simulink model "Hybrid_P2_Parallel_ETE"  (R2017b)
settings: Solver=FixedStepAuto  StartTime=0.0  StopTime=length(Speed)  FixedStep=0.01  MaxStep=0.01  RelTol=1e-3  EnableMultiTasking=on
PostLoadFcn:
  | , if any(exist('dsrtsu_mdlpostloadfcn', 'file') == [2, 3, 6]), try dsrtsu_mdlpostloadfcn('Execute', bdroot); catch fprintf('Error in PostLoadFcn (dsrtsu_mdlpostloadfcn) for model "%s":\n %s\n', bdroot, lasterr); end, end,
undefined symbols (not defined in the file): Actuators, APP1_OOR, APP2_OOR, APP_Mismatch, Brk_Flt, cal, ClutchEngag, CycLength, CycNmb, DiscIntNeverNeededParam, eng, Engine, EngOverTemp, ENGTRQ_MSMCH_Degraded_CP, ENGTRQ_MSMCH_ErrCritical_CP, ENGTRQ_MSMCH_LimpHome_CP, EngTrqMismatch, ess, ESSOverTemp, gb, Gearbox, KeyPos_Flt, lib_Actuators, lib_EMachine_2017a, lib_Sensors_2017a, Loss, LossCAN, Machine, MCUOverTemp, mot, MotDirMismatch, MotOverTemp, MotTrqMismatch, PRNDL_Flt, Ratio, RegenFault, Scope_new, Scopes1, Sensors, Spd, StopIndex, t_amb, time, tloop
libraries: simulink x117, EC2_libraries x9, powerlib_meascontrol x2, CalculationGallon x1, lib_Chassis x1, lib_DCDC x1, lib_Differential x1, lib_HVESS x1, lib_Engine x1, lib_OBC x1, lib_Transmission x1, Transmission_Validation x1
(part 1 of 10)
settings Model: DSRTSU_INTERNAL_RTI_VER=480  DSRTSU_INTERNAL_RTI_TYPE=rti1006  RTICANMMDATA=struct('GeneralSetupData',struct('modelroot','D:\EcoCAR3\Controls\HIL\Y3\P2_Parallel_MIL_Model','generalsettings',struct('filesettings',struct('destfolder',struct('Name','RTICANMM_FILES','Check',1),'buildfolder',struct('Name','.','Check',1),'AbsDestfolder',struct('Name','D:\EcoCAR3\Controls\HIL\Y3\P2_Parallel_MIL_Model\RTICANMM_FILES'),'AbsBuildfolder',struct('Name','D:\EcoCAR3\Controls\HIL\Y3\P2_Parallel_MIL_Model'))),'options',struct('addpaths',1,'rmpaths',1,'addtrcexclusion',logical(1),'cannavigator',struct('checkmonitoring',0),'show_usrtrc',0,'use_usrtrc',0),'advanced',struct('options',[1 1 1 1 1 1 1 1 1 1 1 1 1 1 1 1 1 1 1 1 1 1 1 1 1 1 1 1 1 1 1 1 1 1 1 1 1 1 1 1 1 1 1 1 1 1 1 1 1 1 1 1 1 1 1 1 1 1 1 1 1 1 1 1 1 1 1 1 1 1 1 1 1 1 1 1 1 1 1 1 1 1 1 1 1 1 1 1 1 1 1 1 1 1 1 1 1 1 1 1]),'MPSetup',{{}},'modelname','P2_Parallel_MIL_02_16_2017','block','P2_Parallel_MIL_02_16_2017'))  DSRTSU_INTERNAL_RTIFPGA=70  SimulationMode=accelerator  Creator=EcoCar  LastModifiedBy=Lyu19
settings SolverCC: ExtrapolationOrder=1  NumberNewtonIterations=4
settings OptimizationCC: BlockReduction=off  OptimizeBlockIOStorage=off  BufferReuse=off  GlobalBufferReuse=off  ExpressionFolding=off  LocalBlockOutputs=off  EfficientMapNaN2IntZero=off
settings DebuggingCC: AllowSymbolicDim=off  NonBusSignalsTreatedAsBus=warning  SFUnexpectedBacktrackingDiag=warning  SFNoUnconditionalDefaultTransitionDiag=warning  SFExecutionAtInitializationDiag=none
settings HardwareCC: ProdBitPerPointer=32  ProdBitPerSizeT=32  ProdBitPerPtrDiffT=32  ProdLargestAtomicInteger=Integer  ProdWordSize=32  ProdHWDeviceType=Custom Processor->Custom  TargetBitPerPointer=64  TargetBitPerSizeT=64  TargetBitPerPtrDiffT=64  TargetLongLongMode=on  TargetIntDivRoundTo=Zero  TargetEndianess=LittleEndian  TargetWordSize=64  TargetHWDeviceType=MATLAB Host  ProdEqTarget=off
settings ModelReferenceCC: PropagateSignalLabelsOutOfModel=off
settings CodeAppCC: MaxIdLength=128  StateflowObjectComments=on
settings GRTTargetCC: TargetLangStandard=C89/C90 (ANSI)  CombineOutputUpdateFcns=off  GRTInterface=on
settings ConfigComp: CovMetricSettings=dw  CovHtmlReporting=on  CovSaveCumulativeToWorkspaceVar=on  CovSaveSingleToWorkspaceVar=on  CovExternalEMLEnable=off
settings SimscapeCC: SimscapeNormalizeSystem=off

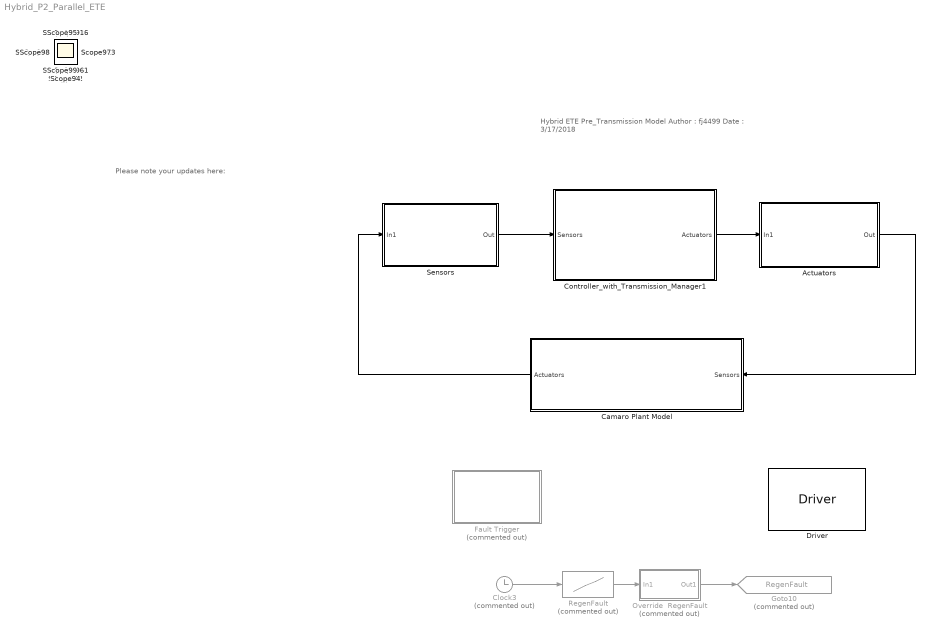
== system Hybrid_P2_Parallel_ETE ==
  note: Please note your updates here:
  note: Hybrid ETE Pre_Transmission Model
      |
      | Author : fj4499
      | Date : 3/17/2018
  Actuators : Subsystem  AncestorBlock=lib_Actuators/Actuators
  Camaro Plant Model : Subsystem
      mask Display: image('Images/Vehicle.jpg')
  Clock3 : Clock  Commented=on
  Controller_with_Transmission_Manager1 : Subsystem
      mask Display: image('Images/HCU.jpg')
  Driver : lib_Driver/Driver  SystemSampleTime=-1
      link override Driver Control/Regen3: Value=0
  "Fault Trigger " : Subsystem  Commented=on  mask(Fault Trigger){Mismatch_APP_ON=on, APP1_OOR_ON=on, APP2_OOR_ON=on, Brk_Flt_ON=on, KeyPos_Flt_ON=on, PRNDL_Flt_ON=on, LossCAN_ON=on, MotTrqMismatch_ON=on, MotDirMismatch_ON=on, EngTrqMismatch_ON=on, MotOverTemp_ON=on, MCUOverTemp_ON=on, EngOverTemp_ON=on, ESSOverTemp_ON=on, ClutchEngagFlt=on}
      mask help:
      | Check the box: override the fault (Control Port value=1;)
      | Uncheck the box: Implement the fault (Control Port value=0;)
      mask DialogControl DriverInterfaceFault Prompt: Driver Interface Fault
      mask DialogControl Container3 Prompt: Component Fault
      mask Display:
      | plot([1 2 2.01 3 4], [0 0 1 1 1]);
      | disp('           Fault Trigger')
  Goto10 : Goto  Commented=on  GotoTag=RegenFault  TagVisibility=global
  Override  RegenFault : Subsystem  Commented=on
  RegenFault : Lookup  Commented=on  InputValues=time  Table=RegenFault  LookUpMeth=Interpolation-Use End Values  OutDataTypeStr=int8
  Sensors : Subsystem  AncestorBlock=lib_Sensors_2017a/Sensors
  Scope{,1..146} (147 alike) : Scope
  wires:
  Clock3/1 -> RegenFault/1
  RegenFault/1 -> Override  RegenFault/1(In1)
  Override  RegenFault/1(Out1) -> Goto10/1
  Controller_with_Transmission_Manager1/1(Actuators) -> Actuators/1(In1)
  Actuators/1(Out) -> Camaro Plant Model/1(Sensors)
  Camaro Plant Model/1(Actuators) -> Sensors/1(In1)
  Sensors/1(Out) -> Controller_with_Transmission_Manager1/1(Sensors)

== system Hybrid_P2_Parallel_ETE/Actuators ==
  In1 : Inport
  Analog : Subsystem
  Bus Creator : BusCreator  Inputs=3
  CAN : Subsystem
  Digital : Subsystem
  Memory : Memory  InheritSampleTime=on
  Out : Outport
  wires:
  In1/1 -> CAN/1(In1), Analog/1(In1), Digital/1(In1)
  Bus Creator/1 -> Memory/1
  Digital/1(Out1) -> Bus Creator/3  "Digital"
  CAN/1(Out1) -> Bus Creator/1  "CAN"
  Analog/1(Out1) -> Bus Creator/2  "Analog"
  Memory/1 -> Out/1

== system Hybrid_P2_Parallel_ETE/Camaro Plant Model ==
  Sensors : Inport
  Add : Sum  Inputs=+++
      mask Display:
      | port_label('input',1,'+');
      | port_label('input',2,'+');
      | port_label('input',3,'+');
  Bus Creator : BusCreator  Inputs=3
  Bus Creator1 : BusCreator  Inputs=7
  Bus Creator2 : BusCreator  Inputs=1
  Bus Selector : BusSelector  OutputSignals=Analog,CAN.to VEH_CAN,CAN.to EBCAN,CAN.to HV_CAN,Digital
  Calculate MPGe : Subsystem  Commented=on
  Calculate MPGe1 : CalculationGallon/Calculate MPGe
  Chassis : lib_Chassis/Chassis  SystemSampleTime=-1
      link override Grade: InputValues=time
  DC-DC Converter : lib_DCDC/DC-DC Converter  SystemSampleTime=-1
  Differential : lib_Differential/Differential  SystemSampleTime=-1
      settings: SourceProductName=The database C:\Users\vrajm\AppData\Roaming\MathWorks\MATLAB\R2017b\slblocks_master.db is locked, or a table in the database is locked. (database is locked)
  E-Machine : Subsystem  AncestorBlock=lib_EMachine_2017a/E-Machine
      mask Display:
      | image('Images/motor.png')
      | color('red');
      | port_label('Input',1,'Volt');
      | port_label('Input',2,'ShaftIn');
      | port_label('Input',3,'SpdOut');
      | port_label('Output',1,'Crr');
      | port_label('Output',2,'ShaftOut');
      | port_label('Output',3,'SpdIn');
  ESS : lib_HVESS/ESS  SystemSampleTime=-1
  Ground : Ground
  ICE Simple1 : lib_Engine/ICE Simple1  SystemSampleTime=-1
  On-Board Charger : lib_OBC/On-Board Charger  SystemSampleTime=-1
      settings: SourceProductName=The database C:\Users\vrajm\AppData\Roaming\MathWorks\MATLAB\R2017b\slblocks_master.db is locked, or a table in the database is locked. (database is locked)
  Scopes : Subsystem  Commented=on
      mask Display: image('Images/Scope.jpg')
  Scopes1 : Subsystem  AncestorBlock=Scope_new/Scopes1
      mask Display: image('Images/Scope.jpg')
  Transmission : Subsystem  AncestorBlock=lib_Transmission/Transmission
      mask Display:
      | image('Images\Trans.png')
      | color('red');
      | port_label('Input',1,'ShaftIn')
      | port_label('Input',2,'SpdOut')
      | port_label('Output',1,'ShaftOut')
      | port_label('Output',2,'SpdIn')
  Transmission Validation Results : Transmission_Validation/Transmission Validation Results  Commented=on  SystemSampleTime=-1
  Wheels : lib_Wheels/Wheels  SystemSampleTime=-1
      link override Grade: InputValues=time
      settings: SourceProductName=The database C:\Users\vrajm\AppData\Roaming\MathWorks\MATLAB\R2017b\slblocks_master.db is locked, or a table in the database is locked. (database is locked)
  Actuators : Outport
  tag scope: Analog=global, Digital=global, HCU_to_EBCAN=global, HCU_to_HV_CAN=global, HCU_to_VEH_CAN=global
  wires:
  Differential/1 -> Wheels/1
  Wheels/1 -> Chassis/1
  Chassis/1 -> Wheels/2
  Differential/2 -> Transmission/2(SpdOut)
  Transmission/1(ShaftOut) -> Differential/1
  ESS/1 -> DC-DC Converter/1, E-Machine/1(voltage), On-Board Charger/1
  DC-DC Converter/1 -> Add/3
  On-Board Charger/1 -> Add/2
  Add/1 -> ESS/1
  Transmission/2(SpdIn) -> E-Machine/3(Mot_SpdOut)
  E-Machine/2(Motor_ShaftOut) -> Transmission/1(ShaftIn)
  E-Machine/1(current) -> Add/1
  Bus Creator/1 -> Actuators/1
  Sensors/1 -> Bus Selector/1
  Bus Selector/1 -> [Analog]  "<Analog>"
  Bus Selector/2 -> [HCU_to_VEH_CAN]  "<to VEH_CAN>"
  Bus Selector/3 -> [HCU_to_EBCAN]  "<to EBCAN>"
  Bus Selector/4 -> [HCU_to_HV_CAN]  "<to HV_CAN>"
  Bus Selector/5 -> [Digital]  "<Digital>"
  Wheels/2 -> Differential/2
  E-Machine/3(Motor_SpdIn) -> ICE Simple1/1
  [ECM_to_HCU] -> Bus Creator1/1
  [TCM_to_HCU] -> Bus Creator1/2
  [BCM_to_HCU] -> Bus Creator1/3
  [BMS_to_HCU] -> Bus Creator1/4
  [MCU_to_HCU] -> Bus Creator1/5
  Bus Creator2/1 -> Bus Creator1/6  "APM_to_HCU"
  [OBC_to_HCU] -> Bus Creator1/7
  Bus Creator1/1 -> Bus Creator/1  "CAN"
  [Driver_Request] -> Bus Creator/2  "Driver_Signals"
  [DCDC_to_HCU] -> Bus Creator/3
  Ground/1 -> Bus Creator2/1  "APM_CAN"
  ICE Simple1/1 -> E-Machine/2(Mot_ShaftIn)

== system Hybrid_P2_Parallel_ETE/Controller_with_Transmission_Manager1 ==
  Sensors : Inport
  HSC : Subsystem
  Actuators : Outport
  wires:
  HSC/1(Actuators) -> Actuators/1
  Sensors/1 -> HSC/1(Sensors)

== system Hybrid_P2_Parallel_ETE/Fault Trigger  ==
  Clock3 : Clock
  Component Diagnostics setting : Subsystem
  Driver Interface Diagnostics setting : Subsystem
  wires:
  Clock3/1 -> Component Diagnostics setting/1(time), Driver Interface Diagnostics setting/1(time)

== system Hybrid_P2_Parallel_ETE/Override  RegenFault ==
  note: This subsystem is used to override the model value of a signal to a constant value
  note: Override Switch Subsystem
  In1 : Inport
  Constant : Constant  Value=0
  Multiport Switch : MultiPortSwitch  DataPortOrder=Zero-based contiguous  Inputs=2
  Signal Override Switch 0 = Use Model 1 = Use Constant : Constant  Value=0
  Out1 : Outport
  wires:
  Signal Override Switch 0 = Use Model 1 = Use Constant/1 -> Multiport Switch/1
  In1/1 -> Multiport Switch/2
  Multiport Switch/1 -> Out1/1
  Constant/1 -> Multiport Switch/3

== system Hybrid_P2_Parallel_ETE/Sensors ==
  In1 : Inport
  Analog : Subsystem
  Bus Creator : BusCreator  Inputs=3
  Bus Selector : BusSelector  OutputSignals=CAN
  CAN : Subsystem
  Digital : Subsystem
  Out : Outport
  wires:
  Bus Creator/1 -> Out/1
  In1/1 -> Digital/1(In1), Analog/1(In1), Bus Selector/1
  Bus Selector/1 -> CAN/1(In1)  "<CAN>"
  CAN/1(Out1) -> Bus Creator/1  "from_CAN"
  Analog/1(Out1) -> Bus Creator/2  "from_Analog"
  Digital/1(Out1) -> Bus Creator/3  "from_Digital"

== system Hybrid_P2_Parallel_ETE/Actuators/Analog ==
  In1 : Inport
  Bus Creator : BusCreator  Inputs=1
  Bus Selector : BusSelector  OutputSignals=Controls.EngAppReq
  Data Type Conversion : DataTypeConversion
  Out1 : Outport
  wires:
  In1/1 -> Bus Selector/1
  Bus Creator/1 -> Out1/1
  Bus Selector/1 -> Data Type Conversion/1  "<EngAppReq>"
  Data Type Conversion/1 -> Bus Creator/1  "EngAppReq"

== system Hybrid_P2_Parallel_ETE/Actuators/CAN ==
  In1 : Inport
  Bus Creator : BusCreator  Inputs=3
  EBCAN : Subsystem
  HV_CAN : Subsystem
  VEH_CAN : Subsystem
  Out1 : Outport
  wires:
  VEH_CAN/1(Out1) -> Bus Creator/1  "to VEH_CAN"
  EBCAN/1(Out1) -> Bus Creator/2  "to EBCAN"
  HV_CAN/1(Out1) -> Bus Creator/3  "to HV_CAN"
  Bus Creator/1 -> Out1/1
  In1/1 -> HV_CAN/1(In1), EBCAN/1(In1), VEH_CAN/1(In1)

== system Hybrid_P2_Parallel_ETE/Actuators/Digital ==
  In1 : Inport
  Bus Creator : BusCreator  Inputs=8
  Bus Selector : BusSelector  OutputSignals=BMS_Digital.T_15,BMS_Digital.T_30,BMS_Digital.T_30C,Fuel_Pump_Control.Pump_Commands.FuelPump_Disable,OBC_Digital.Brusa_Enable,Axiomatic_CAN.GFD_Light,Axiomatic_CAN.HV_Chg_Light,Axiomatic_CAN.Veh_Ready_Light
  Data Type Conversion : DataTypeConversion
  Data Type Conversion1 : DataTypeConversion
  Out1 : Outport
  wires:
  In1/1 -> Bus Selector/1
  Bus Creator/1 -> Out1/1  "Digital"
  Bus Selector/4 -> Bus Creator/4  "<FuelPump_Disable>"
  Bus Selector/3 -> Bus Creator/3  "<T_30C>"
  Bus Selector/2 -> Data Type Conversion1/1  "<T_30>"
  Bus Selector/1 -> Data Type Conversion/1  "<T_15>"
  Bus Selector/5 -> Bus Creator/5  "<Brusa_Enable>"
  Bus Selector/6 -> Bus Creator/6  "<GFD_Light>"
  Bus Selector/7 -> Bus Creator/7  "<HV_Chg_Light>"
  Bus Selector/8 -> Bus Creator/8  "<Veh_Ready_Light>"
  Data Type Conversion/1 -> Bus Creator/1  "T_15"
  Data Type Conversion1/1 -> Bus Creator/2  "T_30"

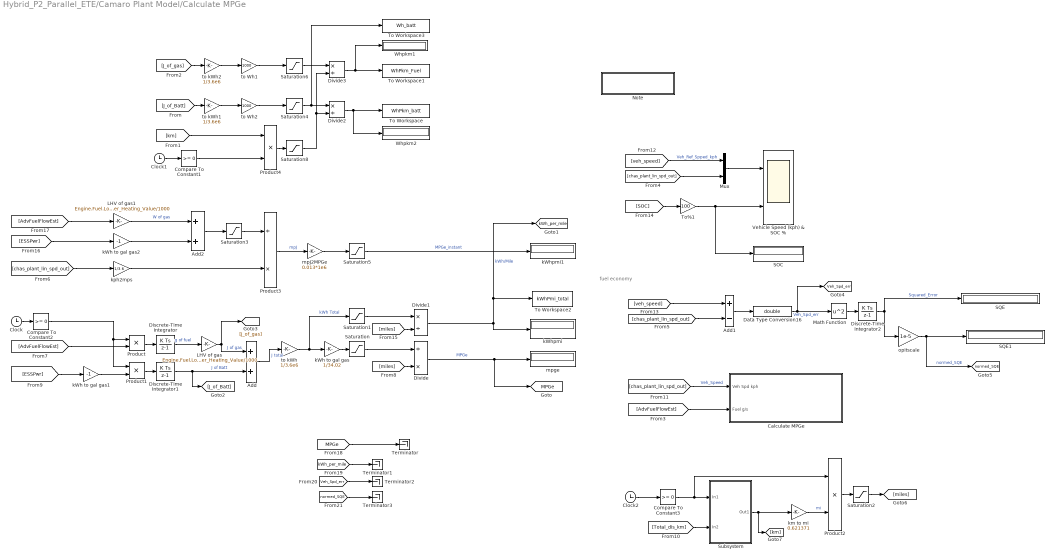
== system Hybrid_P2_Parallel_ETE/Camaro Plant Model/Calculate MPGe ==
  note: fuel economy
  Add : Sum
  Add1 : Sum  Inputs=+-
  Add2 : Sum
  Calculate MPGe : Subsystem
  Clock : Clock
  Clock1 : Clock
  Clock2 : Clock
  Compare To Constant1 : simulink/Logic and Bit Operations/Compare To Constant  relop=>=  const=0  OutDataTypeStr=boolean
  Compare To Constant2 : simulink/Logic and Bit Operations/Compare To Constant  relop=>=  const=0  OutDataTypeStr=boolean
  Compare To Constant3 : simulink/Logic and Bit Operations/Compare To Constant  relop=>=  const=0  OutDataTypeStr=boolean
  Data Type Conversion16 : DataTypeConversion  OutDataTypeStr=double
  Discrete-Time Integrator : DiscreteIntegrator  SampleTime=-1  ICPrevOutput=DiscIntNeverNeededParam  ICPrevScaledInput=DiscIntNeverNeededParam
  Discrete-Time Integrator1 : DiscreteIntegrator  SampleTime=-1  ICPrevOutput=DiscIntNeverNeededParam  ICPrevScaledInput=DiscIntNeverNeededParam
  Discrete-Time Integrator2 : DiscreteIntegrator  SampleTime=-1  ICPrevOutput=DiscIntNeverNeededParam  ICPrevScaledInput=DiscIntNeverNeededParam
  Divide : Product  Inputs=/*
  Divide1 : Product  Inputs=*/
  Divide2 : Product  Inputs=*/
  Divide3 : Product  Inputs=*/
  LHV of gas : Gain  Gain=Engine.Fuel.Lower_Heating_Value/1000
  LHV of gas1 : Gain  Gain=Engine.Fuel.Lower_Heating_Value/1000
  Math Function : Math  Operator=square  SaturateOnIntegerOverflow=on
  Mux : Mux  Inputs=2
  Note : Subsystem
  Product{,1..2,4} (4 alike) : Product
  Product3 : Product  Inputs=/*
  SOC : Display
  SQE : Display
  SQE1 : Display
  Saturation{,1..4,6,8} (7 alike) : Saturate  UpperLimit=inf  LowerLimit=1e-6
  Saturation5 : Saturate  UpperLimit=80  LowerLimit=1e-6
  Subsystem : Subsystem
  Terminator{,1..3} (4 alike) : Terminator
  To Workspace : ToWorkspace  VariableName=WhPkm_batt  SampleTime=-1
  To Workspace1 : ToWorkspace  VariableName=WhPkm_Fuel  SampleTime=-1
  To Workspace2 : ToWorkspace  VariableName=kWhPmi_total  SampleTime=-1
  To Workspace3 : ToWorkspace  VariableName=Wh_batt  SampleTime=-1
  To%1 : Gain  Gain=100
  Vehicle Speed (kph) & SOC % : Scope  NumInputPorts=2
  Whpkm1 : Display
  Whpkm2 : Display
  kWh to gal gas : Gain  Gain=1/34.02
  kWh to gal gas1 : Gain  Gain=-1
  kWh to gal gas2 : Gain  Gain=-1
  kWhpmi : Display
  kWhpmi1 : Display
  km to mi : Gain  Gain=0.621371
  kph2mps : Gain  Gain=1/3.6
  mpJ2MPGe : Gain  Gain=0.013*1e6
  mpge : Display
  opitscale : Gain  Gain=1e-5
  to Wh1 : Gain  Gain=1000
  to Wh2 : Gain  Gain=1000
  to kWh : Gain  Gain=1/3.6e6
  to kWh1 : Gain  Gain=1/3.6e6
  to kWh2 : Gain  Gain=1/3.6e6
  tag scope: MPGe=global, Veh_Spd_err=global, kWh_per_mile=global, normed_SQE=global
  wires:
  Discrete-Time Integrator/1 -> LHV of gas/1  "g of fuel"
  LHV of gas/1 -> Add/1, [J_of_gas]  "J of gas"
  Discrete-Time Integrator1/1 -> Add/2, [J_of_Batt]  "J of Batt"
  Add/1 -> to kWh/1  "J total"
  to kWh/1 -> kWh to gal gas/1, Saturation1/1  "kWh Total"
  km to mi/1 -> Product2/2  "mi"
  kWh to gal gas/1 -> Saturation/1
  Divide/1 -> [MPGe], mpge/1  "MPGe"
  [AdvFuelFlowEst] -> Product/2
  [Total_dis_km] -> Subsystem/2(In2)
  Saturation/1 -> Divide/1
  Saturation1/1 -> Divide1/1
  Divide1/1 -> kWhpmi/1, [kWh_per_mile], To Workspace2/1  "kWh/Mile"
  [veh_speed] -> Mux/1  "Veh_Ref_Spped_kph"
  Mux/1 -> Vehicle Speed (kph) & SOC %/1
  [chas_plant_lin_spd_out] -> Calculate MPGe/1(Veh Spd kph)  "Veh_Speed"
  Discrete-Time Integrator2/1 -> opitscale/1, SQE/1  "Squared_Error"
  Data Type Conversion16/1 -> Math Function/1, [Veh_Spd_err]  "Veh_Spd_err"
  opitscale/1 -> [normed_SQE], SQE1/1  "normed_SQE"
  Math Function/1 -> Discrete-Time Integrator2/1
  Saturation2/1 -> [miles]
  Subsystem/1(Out1) -> km to mi/1, [km]
  Clock/1 -> Compare To Constant2/1
  Product/1 -> Discrete-Time Integrator/1
  Compare To Constant2/1 -> Product1/1, Product/1
  Product1/1 -> Discrete-Time Integrator1/1
  Add1/1 -> Data Type Conversion16/1
  Product2/1 -> Saturation2/1
  LHV of gas1/1 -> Add2/1  "W of gas"
  Product3/1 -> mpJ2MPGe/1  "mpJ"
  mpJ2MPGe/1 -> Saturation5/1
  Add2/1 -> Saturation3/1
  Saturation5/1 -> kWhpmi1/1  "MPGe_instant"
  kph2mps/1 -> Product3/2
  Saturation3/1 -> Product3/1
  [J_of_Batt] -> to kWh1/1
  to kWh1/1 -> to Wh2/1
  to Wh2/1 -> Saturation4/1
  Saturation4/1 -> To Workspace3/1, Divide2/1
  Divide2/1 -> Whpkm2/1, To Workspace/1
  [J_of_gas] -> to kWh2/1
  to kWh2/1 -> to Wh1/1
  to Wh1/1 -> Saturation6/1
  Saturation6/1 -> Divide3/1
  Divide3/1 -> Whpkm1/1, To Workspace1/1
  [km] -> Product4/1
  Product4/1 -> Saturation8/1
  Saturation8/1 -> Divide3/2, Divide2/2
  [ESSPwr] -> kWh to gal gas1/1
  kWh to gal gas1/1 -> Product1/2
  Clock1/1 -> Compare To Constant1/1
  Compare To Constant1/1 -> Product4/2
  [AdvFuelFlowEst] -> Calculate MPGe/2(Fuel g/s)
  [chas_plant_lin_spd_out] -> Add1/2
  [chas_plant_lin_spd_out] -> Mux/2
  [chas_plant_lin_spd_out] -> kph2mps/1
  [veh_speed] -> Add1/1
  [SOC] -> To%1/1
  To%1/1 -> SOC/1, Vehicle Speed (kph) & SOC %/2
  Clock2/1 -> Compare To Constant3/1
  Compare To Constant3/1 -> Product2/1, Subsystem/1(In1)
  [miles] -> Divide/2
  [miles] -> Divide1/2
  [ESSPwr] -> kWh to gal gas2/1
  kWh to gal gas2/1 -> Add2/2
  [AdvFuelFlowEst] -> LHV of gas1/1
  [MPGe] -> Terminator/1
  [kWh_per_mile] -> Terminator1/1
  [Veh_Spd_err] -> Terminator2/1
  [normed_SQE] -> Terminator3/1

== system Hybrid_P2_Parallel_ETE/Camaro Plant Model/E-Machine ==
  voltage : Inport
  Mot_ShaftIn : Inport  Port=2
  Mot_SpdOut : Inport  Port=3
  Clutch Temporary 1 : Subsystem  Commented=on
  IMG Plant : Subsystem
      mask Display:
      | image('Images\Motor.png')
      | color('red');
      | port_label('Input',2,'Volt');
      | port_label('Input',3,'ShaftIn');
      | port_label('Input',4,'SpdOut');
      | port_label('Output',2,'Crr');
      | port_label('Output',3,'ShaftOut');
      | port_label('Output',4,'SpdIn');
  IMG Plant2 : Subsystem  Commented=on
      mask Display:
      | image('Images/motor.png')
      | color('red');
      | port_label('Input',2,'Volt');
      | port_label('Input',3,'SpdOut');
      | port_label('Input',1,'MCU_cmd');
      | port_label('Input',4,'ShaftIn');
      | port_label('Output',1,'Sensor_Out');
      | port_label('Output',2,'Crr');
      | port_label('Output',3,'MotTrqOut');
      | port_label('Output',4,'MotSpdIn');
  Soft MCU : Subsystem
      mask Display: image('SoftECU.jpg')
  current : Outport
  Motor_ShaftOut : Outport  Port=2
  Motor_SpdIn : Outport  Port=3
  tag scope: MCU_to_HCU=global
  wires:
  IMG Plant/2(current) -> current/1
  voltage/1 -> IMG Plant/2(voltage)
  IMG Plant/3(MotShaftOut) -> Motor_ShaftOut/1
  Mot_ShaftIn/1 -> IMG Plant/3(MotShaftIn)
  IMG Plant/1(Out1) -> Soft MCU/2(In1)  "Sensors_to_MCU"
  [HCU_to_HV_CAN] -> Soft MCU/1(In)
  Soft MCU/2(Out1) -> IMG Plant/1("In1 ")  "MCU_to_Actuators"
  Soft MCU/1(Out) -> [MCU_to_HCU]
  Mot_SpdOut/1 -> IMG Plant/4(SpdOut)
  IMG Plant/4(SpdIn) -> Motor_SpdIn/1

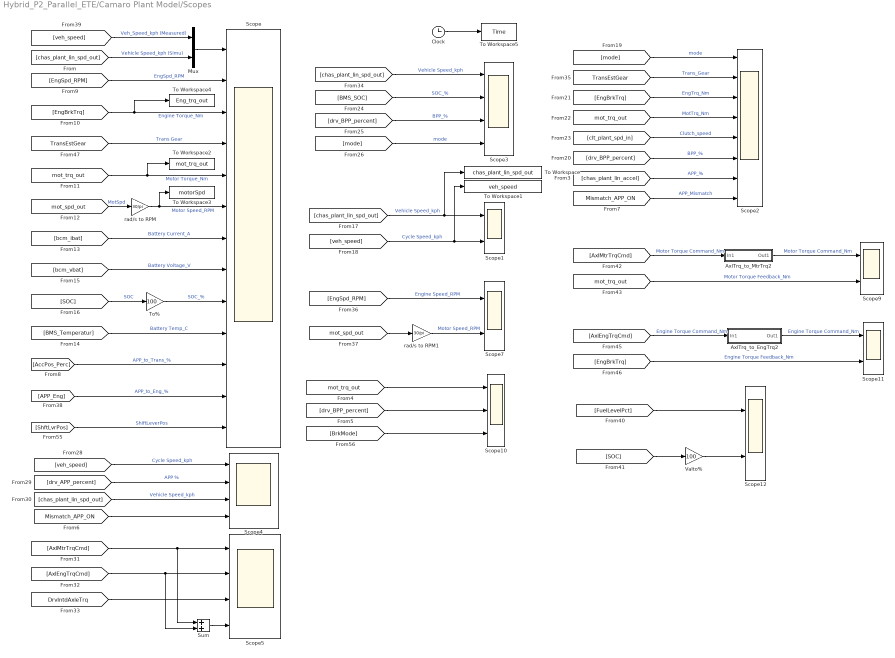
== system Hybrid_P2_Parallel_ETE/Camaro Plant Model/Scopes ==
  AxlTrq_to_EngTrq2 : Subsystem
  AxlTrq_to_MtrTrq2 : Subsystem
  Clock : Clock
      settings: Decimation=WORKSPACE_DECIMATION
  Mux : Mux  Inputs=2
  Scope : Scope  NumInputPorts=13
  Scope{1,7,9,11..12} (5 alike) : Scope  NumInputPorts=2
  Scope10 : Scope  NumInputPorts=3
  Scope2 : Scope  NumInputPorts=8
  Scope3 : Scope  NumInputPorts=4
  Scope4 : Scope  NumInputPorts=4
  Scope5 : Scope  NumInputPorts=4
  Sum : Sum
  To Workspace : ToWorkspace  VariableName=chas_plant_lin_spd_out  SampleTime=-1
  To Workspace1 : ToWorkspace  VariableName=veh_speed  SampleTime=-1
  To Workspace2 : ToWorkspace  VariableName=mot_trq_out  SampleTime=-1
  To Workspace3 : ToWorkspace  VariableName=motorSpd  SampleTime=-1
  To Workspace4 : ToWorkspace  VariableName=Eng_trq_out  SampleTime=-1
  To Workspace5 : ToWorkspace  VariableName=Time  SampleTime=-1
      settings: Decimation=WORKSPACE_DECIMATION
  To% : Gain  Gain=100
  Valto% : Gain  Gain=100
  rad/s to RPM : Gain  Gain=30/pi
  rad/s to RPM1 : Gain  Gain=30/pi
  wires:
  [chas_plant_lin_spd_out] -> Mux/2  "Vehicle Speed_kph (Simu)"
  [EngSpd_RPM] -> Scope/2  "EngSpd_RPM"
  [EngBrkTrq] -> To Workspace4/1, Scope/3  "Engine Torque_Nm"
  [mot_spd_out] -> rad/s to RPM/1  "MotSpd"
  [BMS_Temperatur] -> Scope/10  "Battery Temp_C"
  rad/s to RPM/1 -> To Workspace3/1, Scope/6  "Motor Speed_RPM"
  [mot_trq_out] -> To Workspace2/1, Scope/5  "Motor Torque_Nm"
  To%/1 -> Scope/9  "SOC_%"
  [TransEstGear] -> Scope/4  "Trans Gear"
  [bcm_ibat] -> Scope/7  "Battery Current_A"
  [chas_plant_lin_spd_out] -> Scope3/1  "Vehicle Speed_kph"
  [BMS_SOC] -> Scope3/2  "SOC_%"
  [drv_BPP_percent] -> Scope3/3  "BPP_%"
  [mode] -> Scope3/4  "mode"
  [chas_plant_lin_spd_out] -> To Workspace/1, Scope1/1  "Vehicle Speed_kph"
  [veh_speed] -> To Workspace1/1, Scope1/2  "Cycle Speed_kph"
  [mode] -> Scope2/1  "mode"
  [EngBrkTrq] -> Scope2/3  "EngTrq_Nm"
  [mot_trq_out] -> Scope2/4  "MotTrq_Nm"
  [clt_plant_spd_in] -> Scope2/5  "Clutch_speed"
  [EngSpd_RPM] -> Scope7/1  "Engine Speed_RPM"
  [mot_spd_out] -> rad/s to RPM1/1
  rad/s to RPM1/1 -> Scope7/2  "Motor Speed_RPM"
  [veh_speed] -> Scope4/1  "Cycle Speed_kph"
  [drv_APP_percent] -> Scope4/2  "APP %"
  [chas_plant_lin_spd_out] -> Scope4/3  "Vehicle Speed_kph"
  [AxlMtrTrqCmd] -> Sum/1, Scope5/1
  [AxlEngTrqCmd] -> Sum/2, Scope5/2
  [DrvIntdAxleTrq] -> Scope5/3
  Sum/1 -> Scope5/4
  [AxlMtrTrqCmd] -> AxlTrq_to_MtrTrq2/1(In1)  "Motor Torque Command_Nm"
  [mot_trq_out] -> Scope9/2  "Motor Torque Feedback_Nm"
  [AxlEngTrqCmd] -> AxlTrq_to_EngTrq2/1(In1)  "Engine Torque Command_Nm"
  [EngBrkTrq] -> Scope11/2  "Engine Torque Feedback_Nm"
  [TransEstGear] -> Scope2/2  "Trans_Gear"
  [drv_BPP_percent] -> Scope2/6  "BPP_%"
  [chas_plant_lin_accel] -> Scope2/7  "APP_%"
  AxlTrq_to_MtrTrq2/1(Out1) -> Scope9/1  "Motor Torque Command_Nm"
  AxlTrq_to_EngTrq2/1(Out1) -> Scope11/1  "Engine Torque Command_Nm"
  [bcm_vbat] -> Scope/8  "Battery Voltage_V"
  [Mismatch_APP_ON] -> Scope4/4
  [Mismatch_APP_ON] -> Scope2/8  "APP_Mismatch"
  [SOC] -> To%/1  "SOC"
  [AccPos_Perc] -> Scope/11  "APP_to_Trans_%"
  [APP_Eng] -> Scope/12  "APP_to_Eng_%"
  Mux/1 -> Scope/1
  [veh_speed] -> Mux/1  "Veh_Speed_kph (Measured)"
  Clock/1 -> To Workspace5/1
  [FuelLevelPct] -> Scope12/1
  [SOC] -> Valto%/1
  Valto%/1 -> Scope12/2
  [ShftLvrPos] -> Scope/13  "ShiftLeverPos"
  [mot_trq_out] -> Scope10/1
  [drv_BPP_percent] -> Scope10/2
  [BrkMode] -> Scope10/3

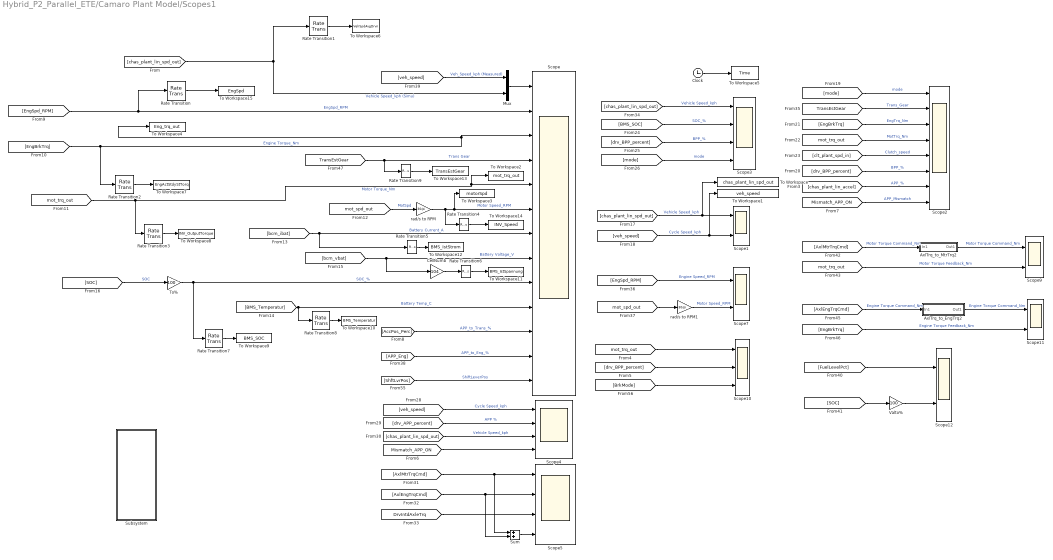
== system Hybrid_P2_Parallel_ETE/Camaro Plant Model/Scopes1 ==
  AxlTrq_to_EngTrq2 : Subsystem
  AxlTrq_to_MtrTrq2 : Subsystem
  CellNumb : Gain  Gain=104
  Clock : Clock
      settings: Decimation=WORKSPACE_DECIMATION
  Mux : Mux  Inputs=2
  Rate Transition{,1..9} (10 alike) : RateTransition  OutPortSampleTime=1
  Scope : Scope  NumInputPorts=13
  Scope{1,7,9,11..12} (5 alike) : Scope  NumInputPorts=2
  Scope10 : Scope  NumInputPorts=3
  Scope2 : Scope  NumInputPorts=8
  Scope3 : Scope  NumInputPorts=4
  Scope4 : Scope  NumInputPorts=4
  Scope5 : Scope  NumInputPorts=4
  Subsystem : Subsystem
  Sum : Sum
  To Workspace : ToWorkspace  VariableName=chas_plant_lin_spd_out  SampleTime=-1
  To Workspace1 : ToWorkspace  VariableName=veh_speed  SampleTime=-1
  To Workspace10 : ToWorkspace  VariableName=BMS_Temperatur  SampleTime=-1
  To Workspace11 : ToWorkspace  VariableName=BMS_IstSpannung  SampleTime=-1
  To Workspace12 : ToWorkspace  VariableName=BMS_IstStrom  SampleTime=-1
  To Workspace13 : ToWorkspace  VariableName=TransEstGear  SampleTime=-1
  To Workspace14 : ToWorkspace  VariableName=INV_Speed  SampleTime=-1
  To Workspace15 : ToWorkspace  VariableName=EngSpd  SampleTime=-1
  To Workspace2 : ToWorkspace  VariableName=mot_trq_out  SampleTime=-1
  To Workspace3 : ToWorkspace  VariableName=motorSpd  SampleTime=-1
  To Workspace4 : ToWorkspace  VariableName=Eng_trq_out  SampleTime=-1
  To Workspace5 : ToWorkspace  VariableName=Time  SampleTime=-1
      settings: Decimation=WORKSPACE_DECIMATION
  To Workspace6 : ToWorkspace  VariableName=VehSpdAvgDrvn  SampleTime=-1
  To Workspace7 : ToWorkspace  VariableName=EngActStdyStTorq  SampleTime=-1
  To Workspace8 : ToWorkspace  VariableName=INV_OutputTorque  SampleTime=-1
  To Workspace9 : ToWorkspace  VariableName=BMS_SOC  SampleTime=-1
  To% : Gain  Gain=100
  Valto% : Gain  Gain=100
  rad/s to RPM : Gain  Gain=30/pi
  rad/s to RPM1 : Gain  Gain=30/pi
  wires:
  Rate Transition9/1 -> To Workspace13/1
  Rate Transition8/1 -> To Workspace10/1
  Rate Transition7/1 -> To Workspace9/1
  Rate Transition6/1 -> To Workspace11/1
  Rate Transition5/1 -> To Workspace12/1
  Rate Transition4/1 -> To Workspace14/1
  Rate Transition3/1 -> To Workspace8/1
  Rate Transition2/1 -> To Workspace7/1
  Rate Transition1/1 -> To Workspace6/1
  Rate Transition/1 -> To Workspace15/1
  CellNumb/1 -> Rate Transition6/1
  [BrkMode] -> Scope10/3
  [drv_BPP_percent] -> Scope10/2
  [mot_trq_out] -> Scope10/1
  [ShftLvrPos] -> Scope/13  "ShiftLeverPos"
  Valto%/1 -> Scope12/2
  [SOC] -> Valto%/1
  [FuelLevelPct] -> Scope12/1
  Clock/1 -> To Workspace5/1
  [veh_speed] -> Mux/1  "Veh_Speed_kph (Measured)"
  Mux/1 -> Scope/1
  [APP_Eng] -> Scope/12  "APP_to_Eng_%"
  [AccPos_Perc] -> Scope/11  "APP_to_Trans_%"
  [SOC] -> To%/1  "SOC"
  [Mismatch_APP_ON] -> Scope2/8  "APP_Mismatch"
  [Mismatch_APP_ON] -> Scope4/4
  [bcm_vbat] -> CellNumb/1, Scope/8  "Battery Voltage_V"
  AxlTrq_to_EngTrq2/1(Out1) -> Scope11/1  "Engine Torque Command_Nm"
  AxlTrq_to_MtrTrq2/1(Out1) -> Scope9/1  "Motor Torque Command_Nm"
  [chas_plant_lin_accel] -> Scope2/7  "APP_%"
  [drv_BPP_percent] -> Scope2/6  "BPP_%"
  [TransEstGear] -> Scope2/2  "Trans_Gear"
  [EngBrkTrq] -> Scope11/2  "Engine Torque Feedback_Nm"
  [AxlEngTrqCmd] -> AxlTrq_to_EngTrq2/1(In1)  "Engine Torque Command_Nm"
  [mot_trq_out] -> Scope9/2  "Motor Torque Feedback_Nm"
  [AxlMtrTrqCmd] -> AxlTrq_to_MtrTrq2/1(In1)  "Motor Torque Command_Nm"
  Sum/1 -> Scope5/4
  [DrvIntdAxleTrq] -> Scope5/3
  [AxlEngTrqCmd] -> Scope5/2, Sum/2
  [AxlMtrTrqCmd] -> Scope5/1, Sum/1
  [chas_plant_lin_spd_out] -> Scope4/3  "Vehicle Speed_kph"
  [drv_APP_percent] -> Scope4/2  "APP %"
  [veh_speed] -> Scope4/1  "Cycle Speed_kph"
  rad/s to RPM1/1 -> Scope7/2  "Motor Speed_RPM"
  [mot_spd_out] -> rad/s to RPM1/1
  [EngSpd_RPM] -> Scope7/1  "Engine Speed_RPM"
  [clt_plant_spd_in] -> Scope2/5  "Clutch_speed"
  [mot_trq_out] -> Scope2/4  "MotTrq_Nm"
  [EngBrkTrq] -> Scope2/3  "EngTrq_Nm"
  [mode] -> Scope2/1  "mode"
  [veh_speed] -> Scope1/2, To Workspace1/1  "Cycle Speed_kph"
  [chas_plant_lin_spd_out] -> Scope1/1, To Workspace/1  "Vehicle Speed_kph"
  [mode] -> Scope3/4  "mode"
  [drv_BPP_percent] -> Scope3/3  "BPP_%"
  [BMS_SOC] -> Scope3/2  "SOC_%"
  [chas_plant_lin_spd_out] -> Scope3/1  "Vehicle Speed_kph"
  [bcm_ibat] -> Scope/7, Rate Transition5/1  "Battery Current_A"
  [TransEstGear] -> Scope/4, Rate Transition9/1  "Trans Gear"
  To%/1 -> Scope/9, Rate Transition7/1  "SOC_%"
  [mot_trq_out] -> Scope/5, To Workspace2/1, Rate Transition3/1  "Motor Torque_Nm"
  rad/s to RPM/1 -> Scope/6, To Workspace3/1, Rate Transition4/1  "Motor Speed_RPM"
  [BMS_Temperatur] -> Scope/10, Rate Transition8/1  "Battery Temp_C"
  [mot_spd_out] -> rad/s to RPM/1  "MotSpd"
  [EngBrkTrq] -> To Workspace4/1, Scope/3, Rate Transition2/1  "Engine Torque_Nm"
  [EngSpd_RPM] -> Scope/2, Rate Transition/1  "EngSpd_RPM"
  [chas_plant_lin_spd_out] -> Mux/2, Rate Transition1/1  "Vehicle Speed_kph (Simu)"

== system Hybrid_P2_Parallel_ETE/Camaro Plant Model/Transmission ==
  ShaftIn : Inport
  SpdOut : Inport  Port=2
  Inputs : Subsystem  AncestorBlock=lib_DCDC/DC-DC Converter/Inputs
  Outputs : Subsystem  AncestorBlock=lib_DCDC/DC-DC Converter/Outputs
  Soft TCM : Subsystem
      mask Display: image('softECU.jpg')
  Transmission Plant : Subsystem
      mask Display:
      | image('Images\Trans.png')
      | color('red');
      | port_label('Input',2,'ShaftIn')
      | port_label('Input',3,'SpdOut')
      | port_label('Output',2,'ShaftOut')
      | port_label('Output',3,'SpdIn')
  ShaftOut : Outport
  SpdIn : Outport  Port=2
  wires:
  Soft TCM/2(Out1) -> Transmission Plant/1("In1 ")  "TCM_to_Actuators"
  Transmission Plant/1(Out1) -> Soft TCM/2(In1)  "Sensors_to_TCM"
  Inputs/1(Inputs) -> Soft TCM/1(In)
  Soft TCM/1(Out) -> Outputs/1(Outputs)
  ShaftIn/1 -> Transmission Plant/2(TorqConvShaftIn)
  SpdOut/1 -> Transmission Plant/3(GearboxSpdOut)
  Transmission Plant/2(GearboxShaftOut) -> ShaftOut/1
  Transmission Plant/3(TorqConvSpdIn) -> SpdIn/1

== system Hybrid_P2_Parallel_ETE/Controller_with_Transmission_Manager1/HSC ==
  Sensors : Inport
  Camaro Fault Detection : Subsystem
  Driver_Requests : Subsystem  RequirementInfo={} %GIDa_7669cec5_5f7d_402f_871c_1fc3f99e6295
  Powertrain Manager : Subsystem
  Actuators : Outport
  wires:
  Driver_Requests/1(DriverRequests) -> Powertrain Manager/2(Driver Request)
  Camaro Fault Detection/1(Diagnostic) -> Driver_Requests/2("Diagnostic "), Powertrain Manager/3(Fault Detection)
  Powertrain Manager/1(Out1) -> Actuators/1
  Sensors/1 -> Driver_Requests/1(Sensors), Powertrain Manager/1(Sensors), Camaro Fault Detection/1(Sensors)
  Powertrain Manager/2(Controls) -> Driver_Requests/3("Controls ")

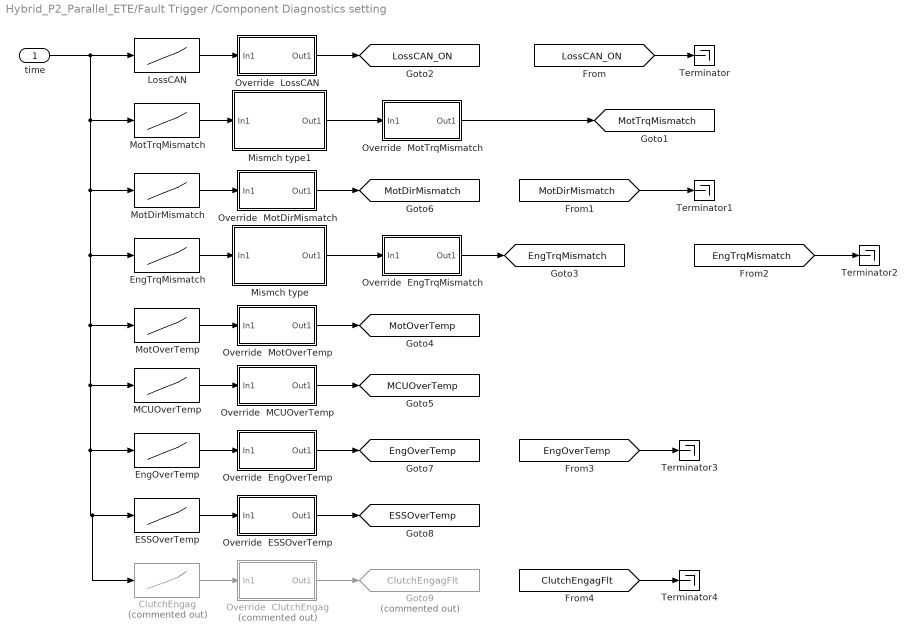
== system Hybrid_P2_Parallel_ETE/Fault Trigger /Component Diagnostics setting ==
  time : Inport
  ClutchEngag : Lookup  Commented=on  InputValues=time  Table=ClutchEngag  LookUpMeth=Interpolation-Use End Values  OutDataTypeStr=int8
  ESSOverTemp : Lookup  InputValues=time  Table=ESSOverTemp  LookUpMeth=Interpolation-Use End Values  OutDataTypeStr=int8
  EngOverTemp : Lookup  InputValues=time  Table=EngOverTemp  LookUpMeth=Interpolation-Use End Values  OutDataTypeStr=int8
  EngTrqMismatch : Lookup  InputValues=time  Table=EngTrqMismatch  LookUpMeth=Interpolation-Use End Values  OutDataTypeStr=int8
  Goto9 : Goto  Commented=on  GotoTag=ClutchEngagFlt  TagVisibility=global
  LossCAN : Lookup  InputValues=time  Table=LossCAN  LookUpMeth=Interpolation-Use End Values  OutDataTypeStr=int8
  MCUOverTemp : Lookup  InputValues=time  Table=MCUOverTemp  LookUpMeth=Interpolation-Use End Values  OutDataTypeStr=int8
  Mismch type : Subsystem
  Mismch type1 : Subsystem
  MotDirMismatch : Lookup  InputValues=time  Table=MotDirMismatch  LookUpMeth=Interpolation-Use End Values  OutDataTypeStr=int8
  MotOverTemp : Lookup  InputValues=time  Table=MotOverTemp  LookUpMeth=Interpolation-Use End Values  OutDataTypeStr=int8
  MotTrqMismatch : Lookup  InputValues=time  Table=MotTrqMismatch  LookUpMeth=Interpolation-Use End Values  OutDataTypeStr=int8
  Override  ClutchEngag : Subsystem  Commented=on
  Override  ESSOverTemp : Subsystem
  Override  EngOverTemp : Subsystem
  Override  EngTrqMismatch : Subsystem
  Override  LossCAN : Subsystem
  Override  MCUOverTemp : Subsystem
  Override  MotDirMismatch : Subsystem
  Override  MotOverTemp : Subsystem
  Override  MotTrqMismatch : Subsystem
  Terminator{,1..4} (5 alike) : Terminator
  tag scope: ESSOverTemp=global, EngOverTemp=global, EngTrqMismatch=global, LossCAN_ON=global, MCUOverTemp=global, MotDirMismatch=global, MotOverTemp=global, MotTrqMismatch=global
  wires:
  MotOverTemp/1 -> Override  MotOverTemp/1(In1)
  LossCAN/1 -> Override  LossCAN/1(In1)
  time/1 -> LossCAN/1, MotTrqMismatch/1, EngTrqMismatch/1, MotOverTemp/1, MCUOverTemp/1, EngOverTemp/1, ClutchEngag/1, ESSOverTemp/1, MotDirMismatch/1
  Override  LossCAN/1(Out1) -> [LossCAN_ON]
  Override  MCUOverTemp/1(Out1) -> [MCUOverTemp]
  Override  EngTrqMismatch/1(Out1) -> [EngTrqMismatch]
  Override  MotDirMismatch/1(Out1) -> [MotDirMismatch]
  MotDirMismatch/1 -> Override  MotDirMismatch/1(In1)
  Override  MotTrqMismatch/1(Out1) -> [MotTrqMismatch]
  MotTrqMismatch/1 -> Mismch type1/1(In1)
  EngTrqMismatch/1 -> Mismch type/1(In1)
  Override  MotOverTemp/1(Out1) -> [MotOverTemp]
  MCUOverTemp/1 -> Override  MCUOverTemp/1(In1)
  Override  EngOverTemp/1(Out1) -> [EngOverTemp]
  EngOverTemp/1 -> Override  EngOverTemp/1(In1)
  Override  ESSOverTemp/1(Out1) -> [ESSOverTemp]
  ESSOverTemp/1 -> Override  ESSOverTemp/1(In1)
  Override  ClutchEngag/1(Out1) -> Goto9/1
  ClutchEngag/1 -> Override  ClutchEngag/1(In1)
  Mismch type/1(Out1) -> Override  EngTrqMismatch/1(In1)
  Mismch type1/1(Out1) -> Override  MotTrqMismatch/1(In1)
  [LossCAN_ON] -> Terminator/1
  [MotDirMismatch] -> Terminator1/1
  [EngTrqMismatch] -> Terminator2/1
  [EngOverTemp] -> Terminator3/1
  [ClutchEngagFlt] -> Terminator4/1

== system Hybrid_P2_Parallel_ETE/Fault Trigger /Driver Interface Diagnostics setting ==
  time : Inport
  APP1_OOR : Lookup  InputValues=time  Table=APP1_OOR  LookUpMeth=Interpolation-Use End Values  OutDataTypeStr=int8
  APP2_OOR : Lookup  InputValues=time  Table=APP2_OOR  LookUpMeth=Interpolation-Use End Values  OutDataTypeStr=int8
  APP_Mismatch : Lookup  InputValues=time  Table=APP_Mismatch  LookUpMeth=Interpolation-Use End Values  OutDataTypeStr=int8
  BPP_Flt : Lookup  InputValues=time  Table=Brk_Flt  LookUpMeth=Interpolation-Use End Values  OutDataTypeStr=int8
  KeyPos_Flt : Lookup  InputValues=time  Table=KeyPos_Flt  LookUpMeth=Interpolation-Use End Values  OutDataTypeStr=int8
  Override  APP1_OOR : Subsystem
  Override  APP2_OOR : Subsystem
  Override  APP_Mismatch : Subsystem
  Override  BPP_Flt : Subsystem
  Override  KeyPos_Flt : Subsystem
  Override  PRNDL_Flt : Subsystem
  PRNDL_Flt : Lookup  InputValues=time  Table=PRNDL_Flt  LookUpMeth=Interpolation-Use End Values  OutDataTypeStr=int8
  Terminator : Terminator
  Terminator1 : Terminator
  tag scope: APP1_OOR_ON=global, APP2_OOR_ON=global, Brk_Flt=global, KeyPos_Flt_ON=global, Mismatch_APP_ON=global, PRNDL_Flt_ON=global
  wires:
  PRNDL_Flt/1 -> Override  PRNDL_Flt/1(In1)
  Override  KeyPos_Flt/1(Out1) -> [KeyPos_Flt_ON]
  BPP_Flt/1 -> Override  BPP_Flt/1(In1)
  APP1_OOR/1 -> Override  APP1_OOR/1(In1)
  Override  APP1_OOR/1(Out1) -> [APP1_OOR_ON]
  APP2_OOR/1 -> Override  APP2_OOR/1(In1)
  Override  APP2_OOR/1(Out1) -> [APP2_OOR_ON]
  Override  BPP_Flt/1(Out1) -> [Brk_Flt]
  Override  PRNDL_Flt/1(Out1) -> [PRNDL_Flt_ON]
  time/1 -> APP_Mismatch/1, APP2_OOR/1, PRNDL_Flt/1, KeyPos_Flt/1, BPP_Flt/1, APP1_OOR/1
  KeyPos_Flt/1 -> Override  KeyPos_Flt/1(In1)
  Override  APP_Mismatch/1(Out1) -> [Mismatch_APP_ON]  "APP_Mismatch"
  APP_Mismatch/1 -> Override  APP_Mismatch/1(In1)
  [APP1_OOR_ON] -> Terminator/1
  [PRNDL_Flt_ON] -> Terminator1/1

== system Hybrid_P2_Parallel_ETE/Sensors/Analog ==
  In1 : Inport
  Bus Creator : BusCreator  Inputs=4
  Bus Selector : BusSelector  OutputSignals=Driver_Signals.drv_APP1,Driver_Signals.drv_APP2,DC_mode,Driver_Signals.Sport_Mode_SW
  Data Type Conversion : DataTypeConversion
  Data Type Conversion1 : DataTypeConversion
  Data Type Conversion2 : DataTypeConversion
  Out1 : Outport
  wires:
  Data Type Conversion/1 -> Bus Creator/3  "DC_mode"
  Data Type Conversion1/1 -> Bus Creator/2  "Driver_APP2"
  Data Type Conversion2/1 -> Bus Creator/1  "Driver_APP1"
  In1/1 -> Bus Selector/1
  Bus Creator/1 -> Out1/1
  Bus Selector/3 -> Data Type Conversion/1  "<DC_mode>"
  Bus Selector/2 -> Data Type Conversion1/1  "<drv_APP2>"
  Bus Selector/1 -> Data Type Conversion2/1  "<drv_APP1>"
  Bus Selector/4 -> Bus Creator/4  "<Sport_Mode_SW>"

== system Hybrid_P2_Parallel_ETE/Sensors/CAN ==
  In1 : Inport
  Bus Creator : BusCreator  Inputs=3
  EBCAN : Subsystem
  HV_CAN : Subsystem
  VEH_CAN : Subsystem
  Out1 : Outport
  wires:
  In1/1 -> VEH_CAN/1(In1), EBCAN/1(In1), HV_CAN/1(In1)
  HV_CAN/1(Out1) -> Bus Creator/3  "fromHV_CAN"
  EBCAN/1(Out1) -> Bus Creator/2  "fromEBCAN"
  Bus Creator/1 -> Out1/1  "from_CAN"
  VEH_CAN/1(Out1) -> Bus Creator/1  "fromVEH_CAN"

== system Hybrid_P2_Parallel_ETE/Sensors/Digital ==
  In1 : Inport
  Bus Creator : BusCreator  Inputs=3
  Bus Selector : BusSelector  OutputSignals=Driver_Signals.SW_Regen_Disable,Driver_Signals.SW_Engine_ON,Driver_Signals.SW_CS_ON
  Data Type Conversion : DataTypeConversion
  Data Type Conversion1 : DataTypeConversion
  Data Type Conversion2 : DataTypeConversion
  Out1 : Outport
  wires:
  In1/1 -> Bus Selector/1
  Bus Selector/1 -> Data Type Conversion1/1  "<SW_Regen_Disable>"
  Bus Selector/2 -> Data Type Conversion/1  "<SW_Engine_ON>"
  Bus Selector/3 -> Data Type Conversion2/1  "<SW_CS_ON>"
  Data Type Conversion/1 -> Bus Creator/2  "SW_Engine_ON"
  Data Type Conversion2/1 -> Bus Creator/3  "SW_CS_ON"
  Data Type Conversion1/1 -> Bus Creator/1  "SW_Regen_Disable"
  Bus Creator/1 -> Out1/1  "Digital"

== system Hybrid_P2_Parallel_ETE/Actuators/CAN/EBCAN ==
  note: BMS_Antrieb
  note: ECM
  In1 : Inport
  Bus Creator : BusCreator  Inputs=7
  Bus Selector : BusSelector  OutputSignals=Controls.EngAppReq,Controls.EngOnReq,Controls.EngTrqCmd,Controls.ShftLvrPos,Controls.SysPwrMd
  Bus Selector1 : BusSelector  OutputSignals=BMS_CAN.ISO_Funktionaler_Req_All,BMS_CAN.ISO_Hybrid_01_Req
  ISO_Hybrid_01_Req : Subsystem
  PPEI_Platform_General_Status : Subsystem
  PPEI_Trans_General_Status_2 : Subsystem
  Out1 : Outport
  wires:
  Bus Creator/1 -> Out1/1
  PPEI_Platform_General_Status/1(Out1) -> Bus Creator/5
  Bus Selector/4 -> PPEI_Trans_General_Status_2/1(In1)  "<ShftLvrPos>"
  Bus Selector/5 -> PPEI_Platform_General_Status/1(In1)  "<SysPwrMd>"
  PPEI_Trans_General_Status_2/1(Out1) -> Bus Creator/4
  Bus Selector/3 -> Bus Creator/3  "<EngTrqCmd>"
  Bus Selector/2 -> Bus Creator/2  "<EngOnReq>"
  Bus Selector/1 -> Bus Creator/1  "<EngAppReq>"
  Bus Selector1/1 -> Bus Creator/6  "<ISO_Funktionaler_Req_All>"
  ISO_Hybrid_01_Req/1(Out1) -> Bus Creator/7
  Bus Selector1/2 -> ISO_Hybrid_01_Req/1(In1)  "<ISO_Hybrid_01_Req>"
  In1/1 -> Bus Selector/1, Bus Selector1/1

== system Hybrid_P2_Parallel_ETE/Actuators/CAN/HV_CAN ==
  In1 : Inport
  Bus Creator : BusCreator  Inputs=4
  Bus Creator1 : BusCreator  Inputs=1
  Bus Creator2 : BusCreator  Inputs=2
  Bus Creator3 : BusCreator  Inputs=5
  Bus Creator5 : BusCreator  Inputs=1
  Bus Selector : BusSelector  OutputSignals=BMS_CAN.MSG_HYB_01.MO_BMS_Sollmodus,Controls.Torque_Command,MCU_CAN.MCU_CAN.VCU_RequestedStateINV,OBC_CAN.NLG5_OC_COM,OBC_CAN.NLG5_OV_COM,OBC_CAN.NLG5_MC_MAX,OBC_CAN.NLG5_C_C_EL,OBC_CAN.NLG5_C_C_EN,MCU_CAN.DCDC_Out.DC_mode
  Data Type Conversion{,1..7} (8 alike) : DataTypeConversion
  Out1 : Outport
  wires:
  Bus Creator/1 -> Out1/1
  In1/1 -> Bus Selector/1
  Bus Selector/1 -> Data Type Conversion/1  "<MO_BMS_Sollmodus>"
  Data Type Conversion/1 -> Bus Creator1/1  "MO_BMS_Sollmodus"
  Bus Creator1/1 -> Bus Creator/1  "MSG_HYB_01"
  Bus Selector/2 -> Data Type Conversion1/1  "<Torque_Command>"
  Bus Selector/3 -> Data Type Conversion2/1  "<VCU_RequestedStateINV>"
  Bus Creator2/1 -> Bus Creator/2  "M192_Command_Message"
  Bus Selector/4 -> Data Type Conversion3/1  "<NLG5_OC_COM>"
  Bus Selector/5 -> Data Type Conversion4/1  "<NLG5_OV_COM>"
  Bus Selector/6 -> Data Type Conversion5/1  "<NLG5_MC_MAX>"
  Bus Selector/7 -> Data Type Conversion6/1  "<NLG5_C_C_EL>"
  Bus Selector/8 -> Data Type Conversion7/1  "<NLG5_C_C_EN>"
  Data Type Conversion1/1 -> Bus Creator2/1  "Torque_Command"
  Data Type Conversion2/1 -> Bus Creator2/2  "Inverter_Enable"
  Bus Creator3/1 -> Bus Creator/3  "NLG5_CTL"
  Data Type Conversion3/1 -> Bus Creator3/1  "NLG5_OC_COM"
  Data Type Conversion4/1 -> Bus Creator3/2  "NLG5_OV_COM"
  Data Type Conversion5/1 -> Bus Creator3/3  "NLG5_MC_MAX"
  Data Type Conversion6/1 -> Bus Creator3/4  "NLG5_C_C_EL"
  Data Type Conversion7/1 -> Bus Creator3/5  "NLG5_C_C_EN"
  Bus Selector/9 -> Bus Creator5/1  "<DC_mode>"
  Bus Creator5/1 -> Bus Creator/4  "DCDC"

== system Hybrid_P2_Parallel_ETE/Actuators/CAN/VEH_CAN ==
  note: TCM
  note: //*Divide the signals out of the Input by component before sending them in the TCM, EBCM etc blocks*//
  In1 : Inport
  BCM : Subsystem  Commented=on
  Bus Creator : BusCreator  Inputs=3
  Bus Creator1 : BusCreator  Inputs=1
  Bus Creator2 : BusCreator  Inputs=1
  Bus Creator3 : BusCreator  Inputs=1
  Bus Selector : BusSelector  OutputSignals=Controls.VehSpdAvgDrvn_kph,Controls.AccPos_Perc
  Data Type Conversion : DataTypeConversion
  Data Type Conversion1 : DataTypeConversion
  Data Type Conversion2 : DataTypeConversion
  EBCM : Subsystem  Commented=on
  Ground1 : Ground  Commented=on
  Ground2 : Ground  Commented=on
  Ground3 : Ground
  Ground4 : Ground  Commented=on
  ICCM : Subsystem  Commented=on
  Terminator : Terminator  Commented=on
  Terminator1 : Terminator  Commented=on
  Terminator2 : Terminator  Commented=on
  Out1 : Outport
  wires:
  ICCM/1(Out1) -> Terminator2/1  "HAct_to_ICCM"
  BCM/1(Out1) -> Terminator/1  "HAct_to_BCM"
  EBCM/1(Out1) -> Terminator1/1  "HAct_to_EBCM"
  Data Type Conversion/1 -> Bus Creator1/1  "VehSpdAvgDrvn"
  Bus Creator/1 -> Out1/1
  Ground1/1 -> EBCM/1(In1)
  Ground2/1 -> ICCM/1(In1)
  Bus Selector/2 -> Data Type Conversion1/1  "<AccPos_Perc>"
  Bus Selector/1 -> Data Type Conversion/1  "<VehSpdAvgDrvn_kph>"
  In1/1 -> Bus Selector/1
  Bus Creator1/1 -> Bus Creator/1  "PPEI_Vehicle_Speed_and_Distance"
  Data Type Conversion1/1 -> Bus Creator2/1  "AccActPos"
  Bus Creator2/1 -> Bus Creator/2  "PPEI_Engine_General_Status_1"
  Bus Creator3/1 -> Bus Creator/3  "ETEI_Engine_General_Status"
  Data Type Conversion2/1 -> Bus Creator3/1  "AccPdlPosPcntFullRng"
  Ground3/1 -> Data Type Conversion2/1
  Ground4/1 -> BCM/1(In1)

== system Hybrid_P2_Parallel_ETE/Camaro Plant Model/Calculate MPGe/Calculate MPGe ==
  Veh Spd kph : Inport
  Fuel g/s : Inport  Port=2
  (L/100 km) : Display
  (MPG) : Display
  (km/L) : Display
  Calculate Fuel Economy : Subsystem
  Goto1 : Goto  Commented=on  GotoTag=km_per_L  TagVisibility=global
  Goto2 : Goto  Commented=on  GotoTag=L_per_100km  TagVisibility=global
  Goto3 : Goto  Commented=on  GotoTag=MPG  TagVisibility=global
  Goto4 : Goto  Commented=on  GotoTag=TotFuel_L  TagVisibility=global
  Total Fuel Used (L) : Display
  wires:
  Fuel g/s/1 -> Calculate Fuel Economy/2(Fuel Flow g/s)
  Calculate Fuel Economy/1(Liter/100Km) -> Goto2/1, (L/100 km)/1  "L/100km"
  Calculate Fuel Economy/3(MPG) -> Goto3/1, (MPG)/1  "MPG"
  Calculate Fuel Economy/4(Fuel Used (L)) -> Goto4/1, Total Fuel Used (L)/1  "TotFuel_L"
  Calculate Fuel Economy/2(Km/Liter) -> (km/L)/1, Goto1/1  "km/L"
  Veh Spd kph/1 -> Calculate Fuel Economy/1(Kph)

== system Hybrid_P2_Parallel_ETE/Camaro Plant Model/Calculate MPGe/Note ==
  note: Note that this is calculating the
      | instantaneous MPGe over time
      | (includes fuel and battery energy used).
      |
      | You should also look at the SOC
      | or energy of the Battery at the end
      | of the cycle, and see what the delta
      | is between the start/end.  If more/less
      | energy is in the Battery at the end, you
      | should determine how you want to
      | account for this difference.  For example,
      | if you consider Plug-In capability to account
      | for energy used, you can factor the cost of
      | plugging in.
      | If you want to assume all energy for this
      | simulation should come from the energy
      | on board the vehicle, then you can make an
      | estimate of how much fuel you would need to
      | use to recharge the batteries using the engine
      | generator set.

== system Hybrid_P2_Parallel_ETE/Camaro Plant Model/Calculate MPGe/Subsystem ==
  In1 : Inport
  In2 : Inport  Port=2
  Add2 : Sum  Inputs=+-
  Switch : Switch  Criteria=u2 > Threshold
  Unit Delay : UnitDelay  SampleTime=-1
  Out1 : Outport
  wires:
  Add2/1 -> Out1/1
  Unit Delay/1 -> Switch/1, Add2/2
  Switch/1 -> Unit Delay/1
  In1/1 -> Switch/2
  In2/1 -> Add2/1, Switch/3

== system Hybrid_P2_Parallel_ETE/Camaro Plant Model/E-Machine/Clutch Temporary 1 ==
  In1 : Inport
  Constant : Constant  Value=0
  Memory : Memory
  Saturation : Saturate  UpperLimit=inf  LowerLimit=0
  Switch : Switch  Criteria=u2 > Threshold
  Out1 : Outport
  wires:
  Switch/1 -> Out1/1
  [cltch] -> Switch/2
  In1/1 -> Saturation/1
  Constant/1 -> Switch/3
  Memory/1 -> Switch/1
  Saturation/1 -> Memory/1

== system Hybrid_P2_Parallel_ETE/Camaro Plant Model/E-Machine/IMG Plant ==
  "In1 " : Inport
  voltage : Inport  Port=2
  MotShaftIn : Inport  Port=3
  SpdOut : Inport  Port=4
  " Actuators" : Subsystem
  Electric Machine : Subsystem
      mask Display:
      | image('Images\Motor.png')
      | color('red');
      | port_label('Input',1,'MotTrqCmd');
      | port_label('Input',2,'Volt');
      | port_label('Input',3,'ShaftIn');
      | port_label('Input',4,'SpdOut');
      | port_label('Output',1,'Crr')
      | port_label('Output',2,'SpdIn')
  Rate Transition7 : RateTransition  OutPortSampleTime=1
  Sensors : Subsystem
  To Workspace1 : ToWorkspace  VariableName=INV_ElectricMachineTemperature  SampleTime=-1
  Out1 : Outport
  current : Outport  Port=2
  MotShaftOut : Outport  Port=3
  SpdIn : Outport  Port=4
  tag scope: DirectionCommand=global, InverterEnabled=global, MotTrqCmd=global
  wires:
  voltage/1 -> Electric Machine/2(voltage2)
  ? -> [LockupCmd]
  [MotTrqCmd] -> Electric Machine/1(MotTrqCmd)
  Electric Machine/1(current) -> current/1
  Electric Machine/2(MotSpdIn1) -> SpdIn/1
  Electric Machine/3(mot_trq_out mot_inertia_out2) -> MotShaftOut/1
  [mot_trq_out] -> Sensors/2(In3)
  Sensors/1(Out1) -> Out1/1
  " Actuators"/1(MotTrqCmd) -> [MotTrqCmd]
  [mot_volt_in] -> Sensors/4(In5)
  "In1 "/1 -> " Actuators"/1(In1)
  [mot_crr_out] -> Sensors/3(In4)
  [mot_temp] -> Rate Transition7/1, Sensors/5(In6)
  " Actuators"/2(DirectionCommand) -> [DirectionCommand]
  " Actuators"/3(InverterEnabled) -> [InverterEnabled]
  [mcu_temp] -> Sensors/6(In1)
  SpdOut/1 -> Electric Machine/4(MotSpdOut)
  MotShaftIn/1 -> Electric Machine/3(mot_trq_in mot_inertia_in)
  [clt_plant_spd_in] -> Sensors/7(In7)
  [mot_spd_out] -> Sensors/1(In2)
  Rate Transition7/1 -> To Workspace1/1
